simulink model "Vb_model"  (R2024b)
settings: Solver=VariableStepAuto  StartTime=0.0  StopTime=100  RelTol=1e-3
settings Model: Creator=shilianshen  LastModifiedBy=shilianshen

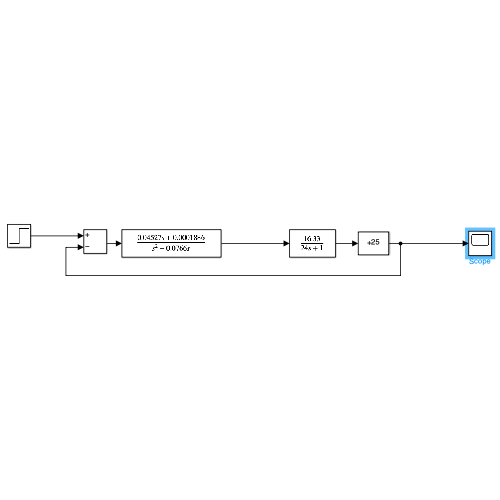
[thumbnail: Simulink's stored preview of the top-level diagram]
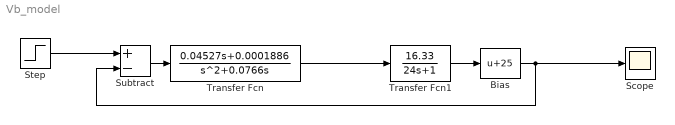
== system Vb_model ==
  Bias : Bias  Bias=25  SaturateOnIntegerOverflow=off
  Scope : Scope
  Step : Step  After=77  SampleTime=0
  Subtract : Sum  Inputs=+-
  Transfer Fcn : TransferFcn  Numerator=[0.04527 0.0001886]  Denominator=[1 0.0766 0]
  Transfer Fcn1 : TransferFcn  Numerator=[16.33]  Denominator=[24 1]
  wires:
  Step/1 -> Subtract/1
  Subtract/1 -> Transfer Fcn/1
  Transfer Fcn/1 -> Transfer Fcn1/1
  Transfer Fcn1/1 -> Bias/1
  Bias/1 -> Subtract/2, Scope/1
